simulink model "AutonomousSteeringSystem"  (R2023a)
settings: Solver=VariableStepAuto  StartTime=0.0  StopTime=15  RelTol=1e-3
libraries: Meldas_library x2, mpclib x1
settings Model: Creator=The MathWorks, Inc.  LastModifiedBy=awear
settings SolverCC: AlgebraicLoopSolver=TrustRegion
settings DataIOCC: ReturnWorkspaceOutputs=off
settings DebuggingCC: UnconnectedInputMsg=warning  UnconnectedOutputMsg=warning  UnconnectedLineMsg=warning  ArithmeticOperatorsInVariantConditions=warning
settings ModelReferenceCC: EnableRefExpFcnMdlSchedulingChecks=on
settings SFSimCC: SimUseLocalCustomCode=off  CustomCodeUndefinedFunction=UseInterfaceOnly
settings RTWCC: RTWUseLocalCustomCode=off
settings CodeAppCC: StateflowObjectComments=on
settings SimscapeCC: SimscapeNormalizeSystem=off

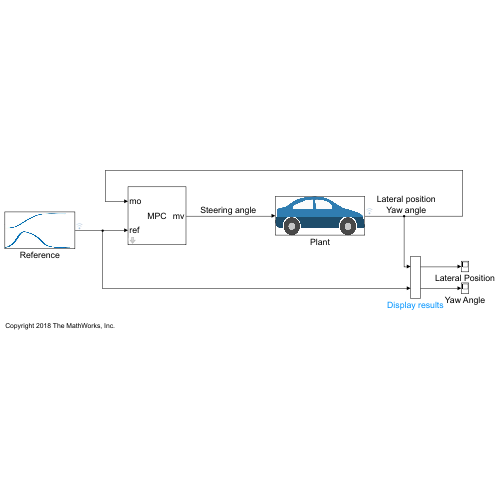
[thumbnail: Simulink's stored preview of the top-level diagram]
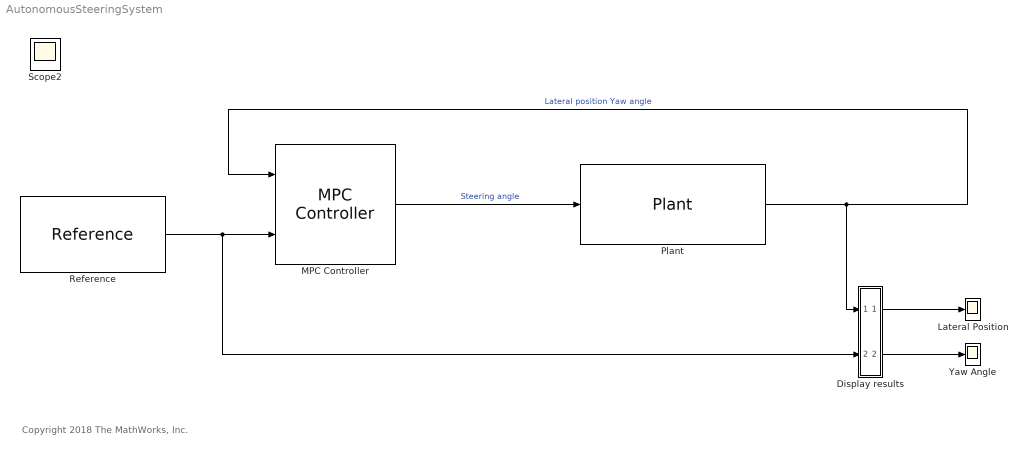
== system AutonomousSteeringSystem ==
  note: Copyright 2018 The MathWorks, Inc.
  Display results : Subsystem
  Lateral Position : Scope
  MPC Controller : mpclib/MPC Controller  SCDEnableBlockLinearizationSpecification=on  mpcobj=mpc1  is_multiple=0  enable_value=0  return_u0=off  updateMPCinCallerWorkspace=on  md_inport=off  mv_inport=off  uref_inport=off  return_cost=off  return_mvseq=off  return_qpstatus=off  return_xseq=off  return_state=off  return_ovseq=off  state_inport=off  umin_inport=off  umax_inport=off  ymin_inport=off  ymax_inport=off  cc_inport=off  ywt_inport=off  uwt_inport=off  duwt_inport=off  rhoeps_inport=off  pm_inport=off  MaximumP=10  HorizonChoice=FixedHorizon  n_ts=0.1  n_p=10  n_mv=1  n_md=0  n_ud=0  n_mo=2  n_uo=0  BlockDataType=double  SampleTimeInherited=off  switch_inport=off
  Plant : Meldas_library/Plant  Vx=15
  Reference : Meldas_library/Reference  SystemSampleTime=-1  VariantActivationTime=update diagram  Latency=0  AutoFrameSizeCalculation=off
  Yaw Angle : Scope
  Scope2 : Scope
  wires:
  MPC Controller/1 -> Plant/1  "Steering angle"
  Plant/1 -> Display results/1(Outputs), MPC Controller/1  "Lateral position Yaw angle"
  Reference/1 -> Display results/2(References), MPC Controller/2
  Display results/2(Out1) -> Yaw Angle/1
  Display results/1(Out2) -> Lateral Position/1

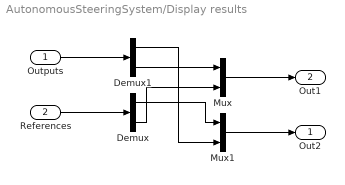
== system AutonomousSteeringSystem/Display results ==
  Outputs : Inport
  References : Inport  Port=2
  Demux : Demux  Outputs=2
  Demux1 : Demux  Outputs=2
  Mux : Mux  Inputs=2
  Mux1 : Mux  Inputs=2
  Out2 : Outport  VectorParamsAs1DForOutWhenUnconnected=off
  Out1 : Outport  Port=2  VectorParamsAs1DForOutWhenUnconnected=off
  wires:
  Demux/2 -> Mux/2
  Mux/1 -> Out1/1
  Demux1/1 -> Mux1/2
  Demux/1 -> Mux1/1
  Demux1/2 -> Mux/1
  Mux1/1 -> Out2/1
  Outputs/1 -> Demux1/1
  References/1 -> Demux/1
